simulink model "fisherman"  (R2014b)
settings: Solver=ode4  StartTime=0.0  StopTime=15  FixedStep=0.01  RelTol=1e-3
values from neighbouring files (symbols this model uses):
  n = input(prompt)    [init.m]    (also in init_consensus.m = 4; init_consensus_15.m = 15; init_mussels.m = 5; init_mussels_2.m = 5)
undefined symbols (not defined in the file or in its folder): vd, X, Y
settings Model: Creator=Demijan  LastModifiedBy=Demijan

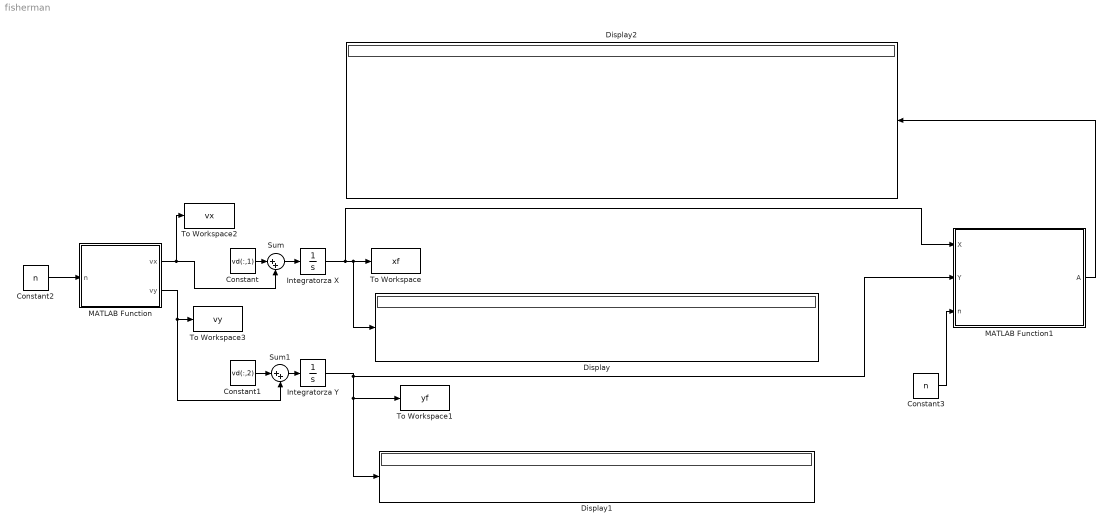
== system fisherman ==
  Constant : Constant  Value=vd(:,1)
  Constant1 : Constant  Value=vd(:,2)
  Constant2 : Constant  Value=n
  Constant3 : Constant  Value=n
  Display : Display
  Display1 : Display
  Display2 : Display
  Integratorza X : Integrator  InitialCondition=X  LimitOutput=on  UpperSaturationLimit=20  LowerSaturationLimit=0
  Integratorza Y : Integrator  InitialCondition=Y  LimitOutput=on  UpperSaturationLimit=20  LowerSaturationLimit=0
  MATLAB Function : MATLAB Function  TreatAsAtomicUnit=on
  MATLAB Function1 : MATLAB Function  TreatAsAtomicUnit=on
  Sum : Sum  Inputs=|++
  Sum1 : Sum  Inputs=|++
  To Workspace : ToWorkspace  VariableName=xf  SaveFormat=Structure  SampleTime=-1
  To Workspace1 : ToWorkspace  VariableName=yf  SaveFormat=Structure  SampleTime=-1
  To Workspace2 : ToWorkspace  VariableName=vx  SaveFormat=Structure  SampleTime=-1
  To Workspace3 : ToWorkspace  VariableName=vy  SaveFormat=Structure  SampleTime=-1
  wires:
  Integratorza Y/1 -> MATLAB Function1/2(Y), To Workspace1/1, Display1/1
  Integratorza X/1 -> MATLAB Function1/1(X), To Workspace/1, Display/1
  Constant/1 -> Sum/1
  Sum/1 -> Integratorza X/1
  Constant1/1 -> Sum1/1
  Sum1/1 -> Integratorza Y/1
  Constant2/1 -> MATLAB Function/1(n)
  MATLAB Function/1(vx) -> To Workspace2/1, Sum/2
  MATLAB Function/2(vy) -> To Workspace3/1, Sum1/2
  Constant3/1 -> MATLAB Function1/3(n)
  MATLAB Function1/1(A) -> Display2/1

== matlab function fisherman/MATLAB Function1 ==
  settings: updateMethod=DISCRETE  sampleTime=0.01
  data: X input; Y input; n input; A output
function A  = fish(X, Y, n)
A=zeros(20,20);
for i=1:n;
    for j=1:n;
        R = sqrt(((X(i)-X(j))^2+(Y(i)-Y(j))^2));
        if R < 4 && i~=j;
            A(i,j)=1;
        else
            A(i,j)=0;
        end
    end
end

== matlab function fisherman/MATLAB Function ==
  settings: updateMethod=DISCRETE  sampleTime=0.01
  data: vx output size=20 [-5..5]; vy output size=20 [-5..5]; n input
function [vx, vy] = fish(n)
vx=zeros(20,1);
vy=zeros(20,1);
for i=1:n;
    vx(i)=4*(rand-0.5);
    vy(i)=4*(rand-0.5);
end
